simulink model "plant_identifier"  (R2019b)
settings: Solver=VariableStepAuto  StartTime=0.0  StopTime=10.0  RelTol=1e-3
settings Model: Creator=admin  LastModifiedBy=IwiLL
settings DebuggingCC: ArithmeticOperatorsInVariantConditions=warning
settings SFSimCC: CustomCodeUndefinedFunction=UseInterfaceOnly

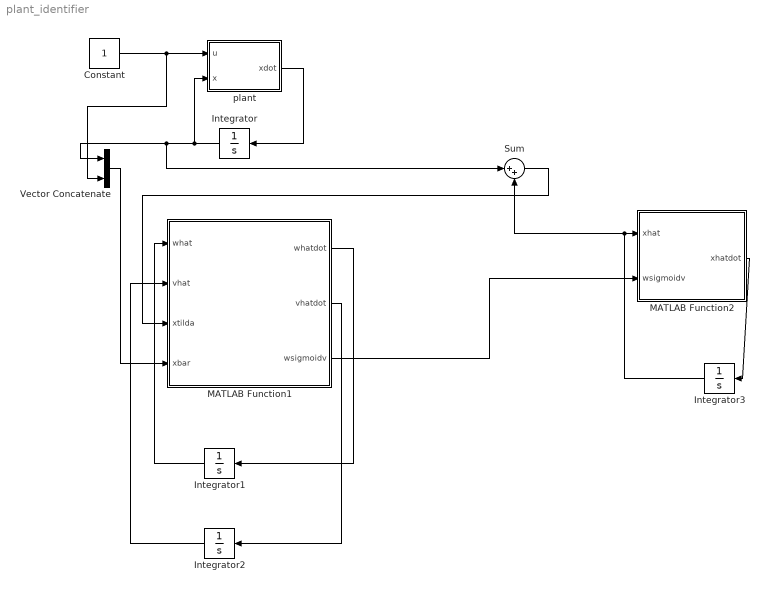
== system plant_identifier ==
  Constant : Constant
  Integrator : Integrator  InitialCondition=zeros(2,1)
  Integrator1 : Integrator  InitialCondition=zeros(2,2)
  Integrator2 : Integrator  InitialCondition=zeros(2,2)
  Integrator3 : Integrator  InitialCondition=zeros(2,1)
  MATLAB Function1 : MATLAB Function  TreatAsAtomicUnit=on
  MATLAB Function2 : MATLAB Function  TreatAsAtomicUnit=on
  Sum : Sum  Inputs=|++
  Vector Concatenate : Concatenate
  plant : MATLAB Function  TreatAsAtomicUnit=on
  wires:
  plant/1(xdot) -> Integrator/1
  Integrator/1 -> Sum/1, Vector Concatenate/1, plant/2(x)
  Constant/1 -> Vector Concatenate/2, plant/1(u)
  MATLAB Function1/1(whatdot) -> Integrator1/1
  Integrator1/1 -> MATLAB Function1/1(what)
  MATLAB Function1/2(vhatdot) -> Integrator2/1
  Integrator2/1 -> MATLAB Function1/2(vhat)
  Vector Concatenate/1 -> MATLAB Function1/4(xbar)
  MATLAB Function2/1(xhatdot) -> Integrator3/1
  Integrator3/1 -> Sum/2, MATLAB Function2/1(xhat)
  MATLAB Function1/3(wsigmoidv) -> MATLAB Function2/2(wsigmoidv)
  Sum/1 -> MATLAB Function1/3(xtilda)

== matlab function plant_identifier/MATLAB Function1 ==
  data: what input; whatdot output; vhat input; xtilda input; xbar input; vhatdot output; wsigmoidv output
function [whatdot,vhatdot,wsigmoidv] = fcn(what,vhat,xtilda,xbar)
 hidden_layer = 2;
 lr1 = 0.1;
 lr2 = 0.1;
 sigmoidvx=zeros(2,1);
 sigmoiddot=zeros(2,1);
 whatdot = zeros(2,2);
 vhatdot = zeros(2,2);
 wsigmoidv = zeros(2,1);
 A = -2*eye(2)
 result = vhat*xbar;
 for i=1:2
     sigmoidvx(i)=sigmoid(result(i))
 end
 sigmoidvxT = transpose(sigmoidvx);
 xtildaT = transpose(xtilda)
 AI = inv(A)
 XTAI = transpose(xtildaT*AI)
 whatdot = -lr1*(XTAI)*(sigmoidvxT)-0.01*what
 for j=1:2
   sigmoiddot(j) = sigmoid(result(j))^2
 end
 hasht=diag(sigmoiddot);
 xbarT=transpose(xbar)
 vhatdot=-lr2*transpose(XTAI*what*(eye(2)-hasht))*xbarT-0.01*vhat
 wsigmoidv = what*(sigmoidvx)
end

== matlab function plant_identifier/plant ==
  data: u input; xdot output; x input
function xdot = fcn(u,x)
xdot=zeros(2,1)
A = [-50,0;1,0];
B = [1;0];
xdot = A*x+B*u;
end

== matlab function plant_identifier/MATLAB Function2 ==
  data: xhat input; xhatdot output; wsigmoidv input
function xhatdot = fcn(xhat,wsigmoidv)
A=-2*eye(2)
xhatdot=A*xhat+wsigmoidv ;
end
